simulink model "rozrusznik"  (R2025b)
settings: Solver=VariableStepAuto  StartTime=0.0  StopTime=10.0  RelTol=1e-3
settings Model: Creator=mintdom  LastModifiedBy=mintdom

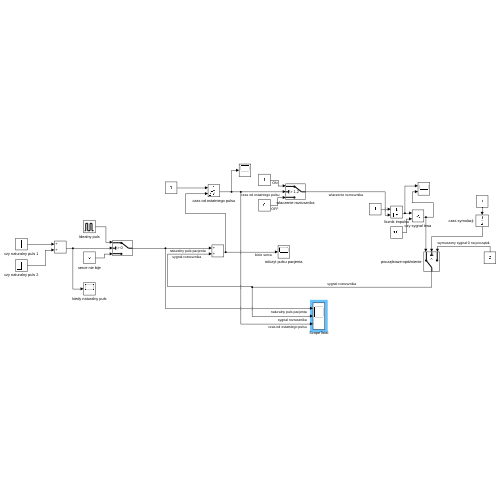
[thumbnail: Simulink's stored preview of the top-level diagram]
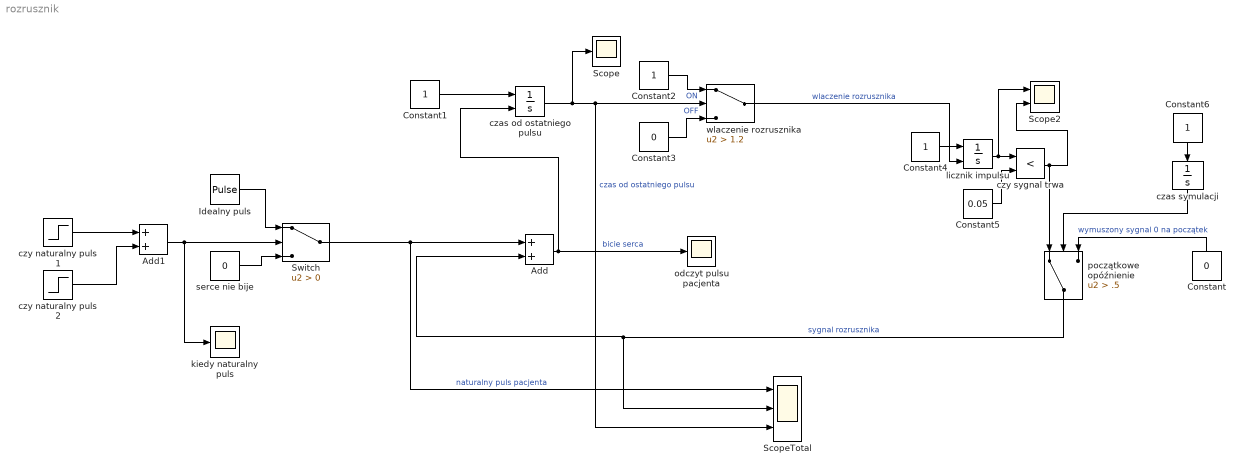
== system rozrusznik ==
  Add : Sum
  Add1 : Sum
  Constant : Constant  Value=0
  Constant{1..2,4,6} (4 alike) : Constant
  Constant3 : Constant  Value=0
  Constant5 : Constant  Value=0.05
  Idealny puls : DiscretePulseGenerator  PulseType=Time based  Period=1  PulseWidth=5
  Scope : Scope
      settings: ActiveDisplayYMinimum=-1  ActiveDisplayYMaximum=1
  Scope2 : Scope  NumInputPorts=2
      settings: ActiveDisplayYMinimum=-1  ActiveDisplayYMaximum=1  DataLoggingVariableName=ScopeData3
  ScopeTotal : Scope  NumInputPorts=3
      settings: ActiveDisplayYMinimum=-0.12499999999999997  ActiveDisplayYMaximum=1.125  DataLoggingVariableName=ScopeData2
  Switch : Switch  Criteria=u2 > Threshold  SaturateOnIntegerOverflow=off  InputSameDT=off
  czas od ostatniego pulsu : Integrator  ExternalReset=rising
  czas symulacji : Integrator
  czy naturalny puls 1 : Step  Time=3.5  Before=1  After=0  SampleTime=0
  czy naturalny puls 2 : Step  Time=7  SampleTime=0
  czy sygnal trwa : RelationalOperator  Operator=<  OutDataTypeStr=boolean  RndMeth=Simplest  InputSameDT=off
  kiedy naturalny puls : Scope
      settings: ActiveDisplayYMinimum=-1  ActiveDisplayYMaximum=1  DataLoggingVariableName=ScopeData4
  licznik impulsu : Integrator  ExternalReset=rising
  odczyt pulsu pacjenta : Scope
      settings: ActiveDisplayYMinimum=0.90830678225944361  ActiveDisplayYMaximum=1.0226222968613818
  początkowe opóźnienie : Switch  Criteria=u2 > Threshold  Threshold=.5  SaturateOnIntegerOverflow=off  InputSameDT=off
  serce nie bije : Constant  Value=0
  wlaczenie rozrusznika : Switch  Criteria=u2 > Threshold  Threshold=1.2  SaturateOnIntegerOverflow=off  InputSameDT=off
  wires:
  Idealny puls/1 -> Switch/1
  serce nie bije/1 -> Switch/3
  Switch/1 -> Add/1, ScopeTotal/1  "naturalny puls pacjenta"
  Constant1/1 -> czas od ostatniego pulsu/1
  czas od ostatniego pulsu/1 -> wlaczenie rozrusznika/2, ScopeTotal/3, Scope/1  "czas od ostatniego pulsu"
  Constant2/1 -> wlaczenie rozrusznika/1  "ON"
  Constant3/1 -> wlaczenie rozrusznika/3  "OFF"
  wlaczenie rozrusznika/1 -> licznik impulsu/2  "wlaczenie rozrusznika"
  Add/1 -> czas od ostatniego pulsu/2, odczyt pulsu pacjenta/1  "bicie serca"
  czy sygnal trwa/1 -> Scope2/2, początkowe opóźnienie/1
  licznik impulsu/1 -> Scope2/1, czy sygnal trwa/1
  Constant5/1 -> czy sygnal trwa/2
  Constant4/1 -> licznik impulsu/1
  czy naturalny puls 1/1 -> Add1/1
  czy naturalny puls 2/1 -> Add1/2
  Add1/1 -> kiedy naturalny puls/1, Switch/2
  Constant6/1 -> czas symulacji/1
  czas symulacji/1 -> początkowe opóźnienie/2
  początkowe opóźnienie/1 -> Add/2, ScopeTotal/2  "sygnal rozrusznika"
  Constant/1 -> początkowe opóźnienie/3  "wymuszony sygnal 0 na początek"
